simulink model "RL"  (R2021a)
settings: Solver=VariableStepAuto  StartTime=0.0  StopTime=100  RelTol=1e-3
settings Model: Creator=Santiago  LastModifiedBy=Santiago

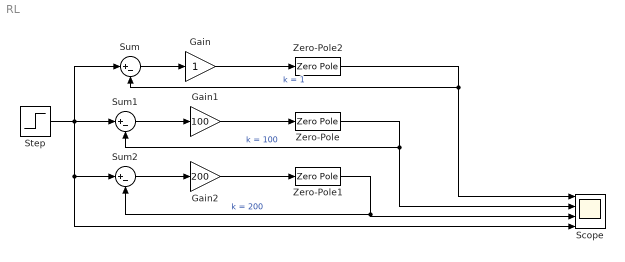
== system RL ==
  Gain : Gain
  Gain1 : Gain  Gain=100
  Gain2 : Gain  Gain=200
  Scope : Scope  NumInputPorts=4
  Step : Step  SampleTime=0
  Sum : Sum  Inputs=|+-
  Sum1 : Sum  Inputs=|+-
  Sum2 : Sum  Inputs=|+-
  Zero-Pole : ZeroPole  Zeros=[-1]  Poles=[0 -2 -4 -4]
  Zero-Pole1 : ZeroPole  Zeros=[-1]  Poles=[0 -2 -4 -4]
  Zero-Pole2 : ZeroPole  Zeros=[-1]  Poles=[0 -2 -4 -4]
  wires:
  Step/1 -> Sum1/1, Sum2/1, Scope/4, Sum/1
  Gain/1 -> Zero-Pole2/1
  Gain1/1 -> Zero-Pole/1
  Gain2/1 -> Zero-Pole1/1
  Zero-Pole2/1 -> Sum/2, Scope/1  "k = 1"
  Zero-Pole/1 -> Sum1/2, Scope/2  "k = 100"
  Zero-Pole1/1 -> Sum2/2, Scope/3  "k = 200"
  Sum/1 -> Gain/1
  Sum1/1 -> Gain1/1
  Sum2/1 -> Gain2/1
